simulink model "jointSpacePDControl"  (R2021a)
settings: Solver=VariableStepAuto  StartTime=0.0  StopTime=5  RelTol=1e-3
values from neighbouring files (symbols this model uses):
  Kd = diag([15, 5, 15])    [assignment6_main.m]
  Kp = diag([40, 30, 80])    [assignment6_main.m]
  q_d = [0.1 pi/3 0.1].'    [assignment6_main.m]
libraries: vrlib x1, simulink x1
settings Model: Creator=fabio  LastModifiedBy=fabio

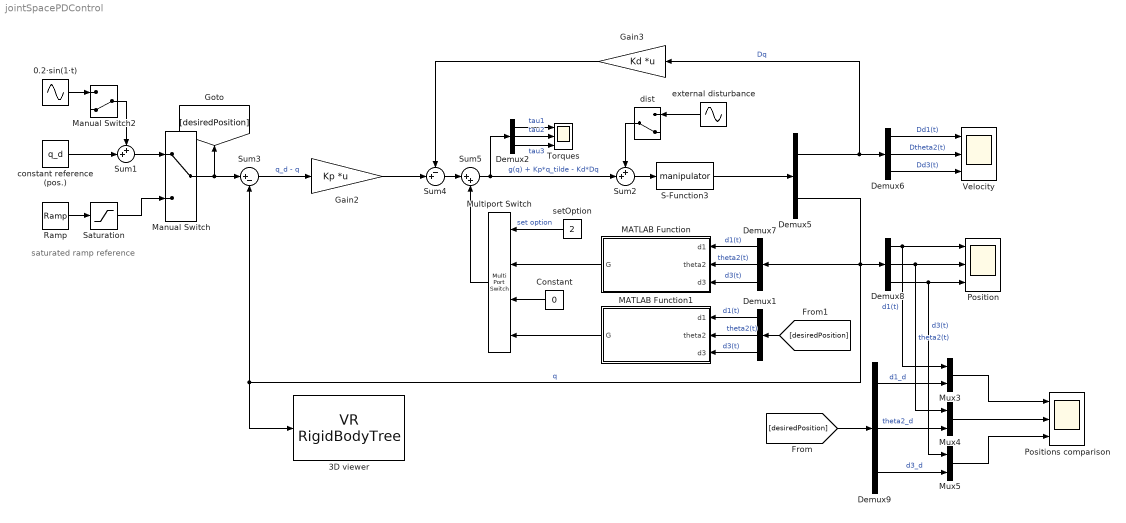
== system jointSpacePDControl ==
  note: saturated ramp reference
  "0.2·sin(1·t) " : Sin  Amplitude=0.2  SampleTime=0
  3D viewer : vrlib/VR RigidBodyTree  RBT=robot  useRBT=off  Ts=0.5  ForceViewerOpen=on
      settings: SourceProductBaseCode=SL
  Constant : Constant  Value=0
  Demux{1..2,6..9} (6 alike) : Demux  Outputs=3
  Demux5 : Demux  Outputs=2
  Gain2 : Gain  Gain=Kp  Multiplication=Matrix(K*u) (u vector)
  Gain3 : Gain  Gain=Kd  Multiplication=Matrix(K*u) (u vector)
  MATLAB Function : MATLAB Function  TreatAsAtomicUnit=on
  MATLAB Function1 : MATLAB Function  TreatAsAtomicUnit=on
  Manual Switch : ManualSwitch
  Manual Switch2 : ManualSwitch  CurrentSetting=0
  Multiport Switch : MultiPortSwitch
  Mux3 : Mux  Inputs=2
  Mux4 : Mux  Inputs=2
  Mux5 : Mux  Inputs=2
  Position : Scope  NumInputPorts=3
  Positions comparison : Scope  NumInputPorts=3
  Ramp : simulink/Sources/Ramp  slope=1  start=0  InitialOutput=0
  S-Function3 : S-Function  FunctionName=manipulator  Parameters=myRobot  SFunctionDeploymentMode=off  EnableBusSupport=off
  Saturation : Saturate  UpperLimit=1.5
  Sum1 : Sum  Inputs=++|
  Sum2 : Sum  Inputs=++|
  Sum3 : Sum  Inputs=|+-
  Sum4 : Sum  Inputs=-+|
  Sum5 : Sum  Inputs=|++
  Torques : Scope  NumInputPorts=3
  Velocity : Scope  NumInputPorts=3
  constant reference (pos.) : Constant  Value=q_d
  dist : ManualSwitch  CurrentSetting=0
  external disturbance : Sin  Amplitude=0.1  SampleTime=0
  setOption : Constant  Value=2
  wires:
  Demux9/2 -> Mux4/2  "theta2_d"
  Mux4/1 -> Positions comparison/2
  Mux3/1 -> Positions comparison/1
  Sum5/1 -> Sum2/2, Demux2/1  "g(q) + Kp*q_tilde - Kd*Dq"
  Demux9/3 -> Mux5/2  "d3_d"
  Sum3/1 -> Gain2/1  "q_d - q"
  Demux9/1 -> Mux3/2  "d1_d"
  Manual Switch/1 -> Sum3/1, [desiredPosition]
  Demux8/2 -> Position/2, Mux4/1  "theta2(t)"
  Sum4/1 -> Sum5/1
  Demux8/3 -> Position/3, Mux5/1  "d3(t)"
  Demux6/3 -> Velocity/3  "Dd3(t)"
  Demux6/2 -> Velocity/2  "Dtheta2(t)"
  Demux6/1 -> Velocity/1  "Dd1(t)"
  S-Function3/1 -> Demux5/1
  Demux8/1 -> Position/1, Mux3/1  "d1(t)"
  Gain3/1 -> Sum4/1
  Gain2/1 -> Sum4/2
  Mux5/1 -> Positions comparison/3
  Demux7/1 -> MATLAB Function/1(d1)  "d1(t)"
  Demux7/2 -> MATLAB Function/2(theta2)  "theta2(t)"
  Demux7/3 -> MATLAB Function/3(d3)  "d3(t)"
  Multiport Switch/1 -> Sum5/2
  Demux1/3 -> MATLAB Function1/3(d3)  "d3(t)"
  Demux1/2 -> MATLAB Function1/2(theta2)  "theta2(t)"
  Demux1/1 -> MATLAB Function1/1(d1)  "d1(t)"
  [desiredPosition] -> Demux1/1
  MATLAB Function1/1(G) -> Multiport Switch/4
  MATLAB Function/1(G) -> Multiport Switch/2
  Constant/1 -> Multiport Switch/3
  setOption/1 -> Multiport Switch/1  "set option"
  Demux5/1 -> Demux6/1, Gain3/1  "Dq"
  Demux5/2 -> Demux8/1, Demux7/1, 3D viewer/1, Sum3/2  "q"
  constant reference (pos.)/1 -> Sum1/2
  Sum1/1 -> Manual Switch/1
  Saturation/1 -> Manual Switch/2
  Ramp/1 -> Saturation/1
  Demux2/1 -> Torques/1  "tau1"
  Demux2/2 -> Torques/2  "tau2"
  Demux2/3 -> Torques/3  "tau3"
  Sum2/1 -> S-Function3/1
  external disturbance/1 -> dist/1
  dist/1 -> Sum2/1
  "0.2·sin(1·t) "/1 -> Manual Switch2/1
  Manual Switch2/1 -> Sum1/1
  [desiredPosition] -> Demux9/1

== matlab function jointSpacePDControl/MATLAB Function ==
  data: d1 input; G output; theta2 input; d3 input
function G = gravityTerm(d1, theta2, d3) 
    q = [d1 theta2 d3];
    G = get_G_matrix(q);
end

== matlab function jointSpacePDControl/MATLAB Function1 ==
  data: d1 input; G output; theta2 input; d3 input
function G = gravityTerm(d1, theta2, d3) 
    q = [d1 theta2 d3];
    G = get_G_matrix(q);
end
